simulink model "nonLin_Model_plantOnly"  (R2023b)
settings: Solver=VariableStepAuto  StartTime=0.0  StopTime=7  FixedStep=Ts  MaxStep=0.002  RelTol=1e-3
InitFcn:
  | sysParam = load("sysParam.mat");
  | load('./zz_temp/controlletTypeToUse.mat')
settings Model: Creator=maxja  LastModifiedBy=maxja

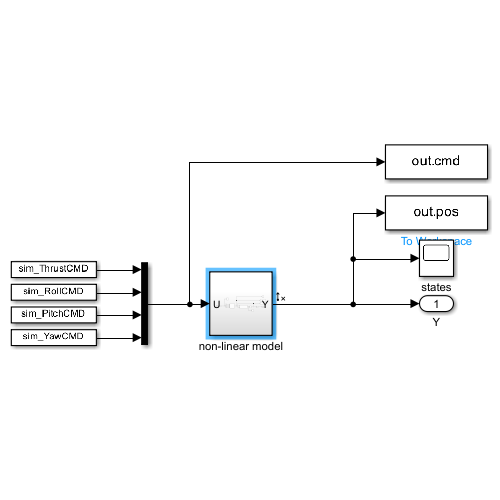
[thumbnail: Simulink's stored preview of the top-level diagram]
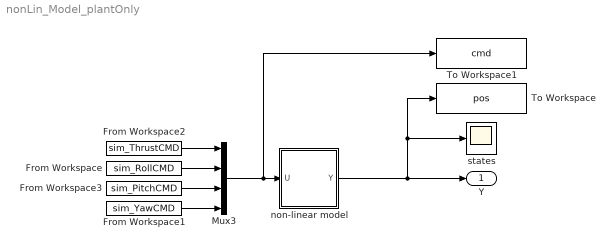
== system nonLin_Model_plantOnly ==
  From Workspace : FromWorkspace  VariableName=sim_RollCMD
  From Workspace1 : FromWorkspace  VariableName=sim_YawCMD
  From Workspace2 : FromWorkspace  VariableName=sim_ThrustCMD
  From Workspace3 : FromWorkspace  VariableName=sim_PitchCMD
  Mux3 : Mux
  To Workspace : ToWorkspace  VariableName=pos  SaveFormat=Timeseries  SampleTime=-1
  To Workspace1 : ToWorkspace  VariableName=cmd  SaveFormat=Timeseries  SampleTime=-1
  non-linear model : Subsystem
  states : Scope
  Y : Outport
  wires:
  non-linear model/1(Y) -> To Workspace/1, states/1, Y/1
  From Workspace2/1 -> Mux3/1
  From Workspace/1 -> Mux3/2
  From Workspace3/1 -> Mux3/3
  Mux3/1 -> To Workspace1/1, non-linear model/1(U)
  From Workspace1/1 -> Mux3/4

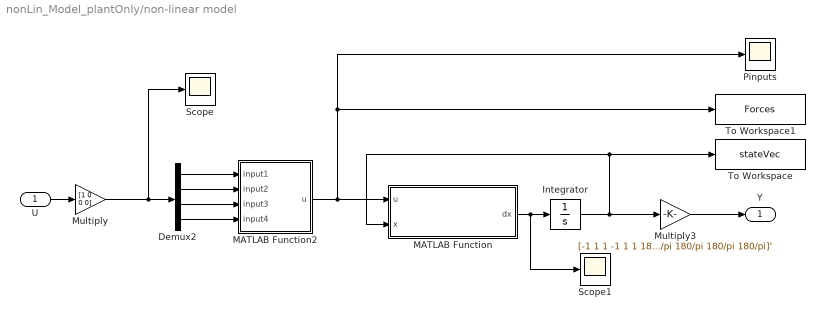
== system nonLin_Model_plantOnly/non-linear model ==
  U : Inport  PortDimensions=4
  Demux2 : Demux
  Integrator : Integrator  InitialCondition=[0;0;0;0;0;0;0;0;0;0;0;0]
  MATLAB Function : MATLAB Function  TreatAsAtomicUnit=on
  MATLAB Function2 : MATLAB Function  TreatAsAtomicUnit=on
  Multiply : Gain  Gain=[1 0 0 0]
  Multiply3 : Gain  Gain=[-1 1 1 -1 1 1 180/pi 180/pi 180/pi 180/pi 180/pi 180/pi]'
  Pinputs : Scope
  Scope : Scope
  Scope1 : Scope
  To Workspace : ToWorkspace  VariableName=stateVec  SaveFormat=Timeseries  SampleTime=-1
  To Workspace1 : ToWorkspace  VariableName=Forces  SaveFormat=Timeseries  SampleTime=-1
  Y : Outport
  wires:
  MATLAB Function/1(dx) -> Scope1/1, Integrator/1
  MATLAB Function2/1(u) -> Pinputs/1, To Workspace1/1, MATLAB Function/1(u)
  Demux2/2 -> MATLAB Function2/2(input2)
  Demux2/1 -> MATLAB Function2/1(input1)
  Demux2/3 -> MATLAB Function2/3(input3)
  Demux2/4 -> MATLAB Function2/4(input4)
  Integrator/1 -> Multiply3/1, To Workspace/1, MATLAB Function/2(x)
  Multiply3/1 -> Y/1
  U/1 -> Multiply/1
  Multiply/1 -> Scope/1, Demux2/1

== matlab function nonLin_Model_plantOnly/non-linear model/MATLAB Function ==
  data: u input; dx output; x input; sysParam parameter
function dx= nonLinDrone(u,x, sysParam)
    m = 0.03639;%sysParam.m;
    I = sysParam.I;
    g = sysParam.g;
    invI = sysParam.invI;
    L = sysParam.L;
    % L = 0.048;% Distance from center of mass to rotors

    dx = zeros(12,1);
    
    % Angle states for easier use
    phi   = x(7); 
    theta = x(8); 
    psi   = x(9);
    p     = x(10); 
    q     = x(11); 
    r     = x(12);

    % Rotation matrix
    R = rotation_matrix(phi, theta, psi);

    % x and xdot definition
    dx(1:3,1) = [x(4); x(5); x(6)];
    dx(4:6,1) = 1/m*([0;0;-m*g]+R*[0;0;u(1)]);

    multiplication_matrix_pqr = ([1 sin(phi)*tan(theta) cos(phi)*tan(theta);0 cos(phi) -sin(phi);0 sin(phi)/cos(theta) cos(phi)/cos(theta)]);

    dx(7:9,1) = multiplication_matrix_pqr*[p;q;r];
    dx(10:12,1) = invI * ([u(2); u(3); u(4)] - cross([x(10);x(11);x(12)],I*[x(10);x(11);x(12)]));

function R = rotation_matrix(phi, theta, psi)
    R_x = [1 0 0; 0 cos(phi) -sin(phi); 0 sin(phi) cos(phi)];
    R_y = [cos(theta) 0 sin(theta); 0 1 0; -sin(theta) 0 cos(theta)];
    R_z = [cos(psi) -sin(psi) 0; sin(psi) cos(psi) 0; 0 0 1];

    R = R_z * R_y * R_x;
end
end

== matlab function nonLin_Model_plantOnly/non-linear model/MATLAB Function2 ==
  data: input1 input; u output; input2 input; input3 input; input4 input
function u = fcn(input1,input2,input3,input4)

L = 0.048;% Distance from center of mass to rotors
% syms Thrust controlRoll controlPitch controlYaw
% 
% inputs = [Thrust;
%           controlRoll;
%           controlPitch;
%           controlYaw];

cmdi = [1 -0.5  0.5  1;
        1 -0.5 -0.5 -1;
        1  0.5 -0.5  1;
        1  0.5  0.5 -1]*[input1;input2;input3;input4];
% cmdi = [1 -2  2  1;
%         1 -2 -2 -1;
%         1  2 -2  1;
%         1  2  2 -1]*[input1;input2;input3;input4]

Kf2 = 2.130295e-11;
Kf1 = 1.032633e-6;
Kf0 = 5.484560e-4;

Km1 = 0.005964552;
Km0 = 1.563383;

Fi = Kf2*cmdi.^2+Kf1*cmdi+Kf0;
Mi = Km1*Fi+Km0;

u1 = sum(Fi);
u2 = sqrt(2)*L*((Fi(1)+Fi(2))-(Fi(3)+Fi(4)));
u3 = sqrt(2)*L*((Fi(2)+Fi(3))-(Fi(1)+Fi(4)));
% u2 = L*(Fi(2)-Fi(4));
% u3 = L*(Fi(3)-Fi(1));
u4 = Mi(1)-Mi(2)+Mi(3)-Mi(4);

u = [u1;u2;u3;u4];

end
